simulink model "vanderpol"  (R2022b)
settings: Solver=ode5  StartTime=0.0  StopTime=7  FixedStep=0.01  RelTol=1e-3
settings Model: Creator=b6062805  LastModifiedBy=b6062805
settings DataIOCC: SaveFormat=Structure  SignalLogging=off  DSMLogging=off  ReturnWorkspaceOutputs=off

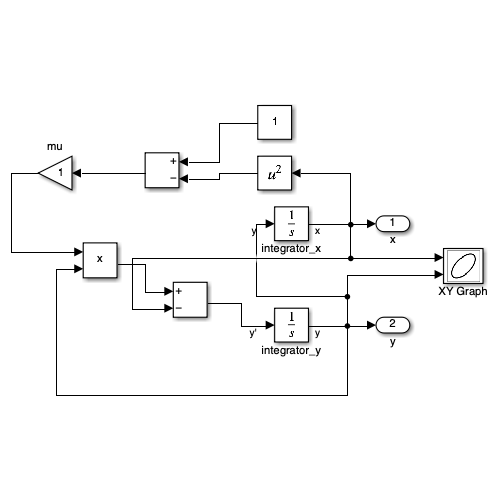
[thumbnail: Simulink's stored preview of the top-level diagram]
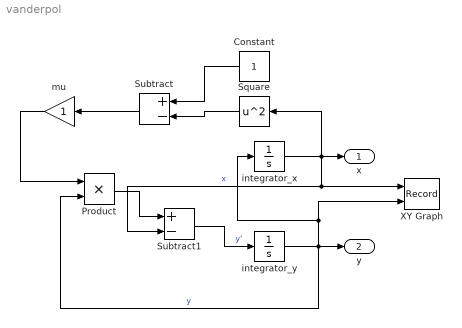
== system vanderpol ==
  Constant : Constant
  Product : Product
  Square : Math  Operator=square
  Subtract : Sum  Inputs=+-
  Subtract1 : Sum  Inputs=+-
  XY Graph : Record  FileSettingsInternal="{\"entries\":[{\"content\":{\"excelSettings\":{\"content\":{},\"type\":\"Streamout.ExcelSettings\"}},\"type\":\"Streamout.FileSettingStorage\",\"uuid\":\"93645cb5-39d6-4b5f-bff2-ad29d9c7d749\"}],\"packageUris\":[\"http://schema.mathworks.com/mf0/streamout_blocks/R2020a\"],\"version\":\"1.0\"}"  Layout=[1 1]  SignalsInternal="{\"entries\":[{\"content\":{\"signals\":[{\"content\":{\"blockPath\":[\"vanderpol/XY Graph\"],\"channel\":[],\"dimensions\":[1],\"domain\":\"vanderpol/XY Graph\",\"lineColor\":\"#a2142f\",\"plots\":[1],\"port\":1,\"sid\":[],\"signalID\":396,\"signalName\":\"x\"},\"type\":\"RecordBlkView.Signal\",\"uuid\":\"90e3f62e-15e3-4100-9f80-cf312a494c78\"},{\"content\":{\"blockPath\":[\"vanderpol/XY Graph\"],\"channel\":[],\"dimensions\":[1],\"domain\":\"vanderpol/XY Graph\",\"lineColor\":\"#139fff\",\"plots\":[1],\"port\":2,\"sid\":[],\"signalID\":399,\"signalName\":\"y\"},\"type\":\"RecordBlkView.Signal\",\"uuid\":\"73fa060b-3a6f-4c9f-b527-f0f8a39b39df\"}]},\"type\":\"RecordBlkView.InputSignals\",\"uuid\":\"16cb959e-9d4e-4fa5-895f-3582522ee266\"}],\"packageUris\":[\"http://schema.mathworks.com/mf0/streamout_blocks/R2020a\"],\"version\":\"1.0\"}"  VisualizationBindings="{\"xyplotplugin\":{\"info\":[{\"series\":[{\"bindingParametersList\":[{\"parameter\":\"X-Axis\",\"signalID\":396,\"signalName\":\"x\"},{\"parameter\":\"Y-Axis\",\"signalID\":399,\"signalName\":\"y\"}],\"seriesID\":45501}],\"subplotID\":1}]}}"  CompatibilityTag=XY
  integrator_x : Integrator  InitialCondition=1.25
  integrator_y : Integrator  InitialCondition=2.25
  mu : Gain
  x : Outport
  y : Outport  Port=2
  wires:
  integrator_x/1 -> XY Graph/1, Subtract1/2, x/1, Square/1  "x"
  integrator_y/1 -> y/1, XY Graph/2, integrator_x/1, Product/2  "y"
  Square/1 -> Subtract/2
  Constant/1 -> Subtract/1
  Subtract/1 -> mu/1
  mu/1 -> Product/1
  Product/1 -> Subtract1/1
  Subtract1/1 -> integrator_y/1  "y'"
